simulink model "Opticflowtest"  (Simulink 7.6)
settings: Solver=ode45  StartTime=0.0  StopTime=inf  RelTol=1e-3
undefined symbols (not defined in the file or in its folder): Horn, none, Schunck, videoinput
libraries: imaqlib x1, dspstat3 x1, vipanalysis x1, simulink x1
settings Model: Creator=pacifist  LastModifiedBy=pacifist

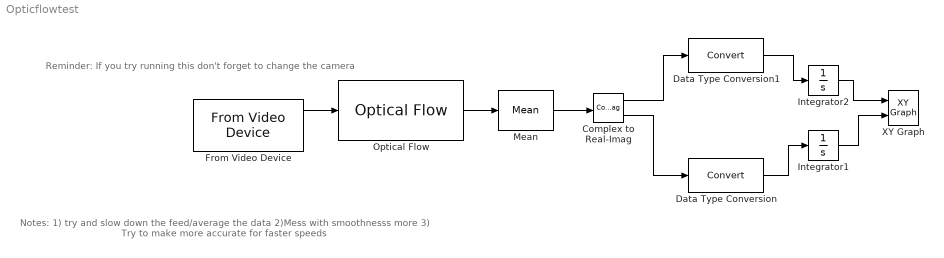
== system Opticflowtest ==
  note: Notes:
      | 1) try and slow down the feed/average the data
      | 2)Mess with smoothnesss more
      | 3) Try to make more accurate for faster speeds
  note: Reminder:
      | If you try running this don't forget to change the camera
  Complex to Real-Imag : ComplexToRealImag
  Data Type Conversion : DataTypeConversion
  Data Type Conversion1 : DataTypeConversion
  From Video Device : imaqlib/From Video Device  DialogController=imaqcreatedialog  DialogControllerArgs=DataTag1  DeviceMenu=linuxvideo 1 (UVC Camera (046d:0804))  Device=linuxvideo 1 (UVC Camera (046d:0804))  ObjConstructor=videoinput('linuxvideo', 1)  VideoFormatMenu=YUYV_160x120  VideoFormat=YUYV_160x120  VideoSource=Camera 1  ROIPosition=[0 0 120 160]  EnableHWTrigger=off  TriggerConfiguration=none/none  SampleTime=1/30  OutputPortsMode=Separate color signals  DataType=single  CanDoHWTrigger=no  ReturnedColorSpace=YCbCr  BlockHandle=2231.0004  ROIWidth=160  ROIHeight=120  ROIColumn=0  ROIRow=0  EngXMLPath=/usr/local/MATLAB/R2010b/toolbox/imaq/imaq/private  DevXMLPath=/usr/local/MATLAB/R2010b/toolbox/imaq/imaqadaptors/glnx86  EngLibPath=/usr/local/MATLAB/R2010b/toolbox/imaq/imaqblks/imaqmex/glnx86
  Integrator1 : Integrator  LimitOutput=on  UpperSaturationLimit=.01  LowerSaturationLimit=-.01
  Integrator2 : Integrator  LimitOutput=on  UpperSaturationLimit=.01  LowerSaturationLimit=-.01
  Mean : dspstat3/Mean  DialogController=dspDDGCreate  DialogControllerArgs=DataTag3  run=off  reset_popup=None  directionMode=Entire input  dimension=1  treatSBRowAsCol=on  roiEnable=off  roiType=Rectangles  roiPortion=Entire ROI  roiOutput=Individual statistics for each ROI  roiFlag=off  outputDataTypeStr=Inherit: Same as accumulator  outputLastDataTypeStr=Inherit: Same as accumulator  outputMin=[]  outputMax=[]  accumMode=Binary point scaling  accumWordLength=32  accumFracLength=0  accumDataTypeStr=fixdt([],32,0)  accumLastDataTypeStr=fixdt([],32,0)  roundingMode=Floor  overflowMode=off
  Optical Flow : vipanalysis/Optical Flow  DialogController=vipDDGCreate  DialogControllerArgs=DataTag4  SystemSampleTime=-1  method=Horn-Schunck  gradMethod=Difference filter [-1 1]  which2img=Current frame and N-th frame back  N=1  outVelForm=Horizontal and vertical components in complex form  lambda=5  stop_criteria=When maximum number of iterations is reached  maxAllowAbsDiff=eps  maxIter=10  numInports=3  sigmaS=1.5  sigmaW=1  eigTh=0.0039  discardNormalFlow=off  outputCurrentImage=off  prodOutputMode=Binary point scaling  prodOutputWordLength=32  prodOutputFracLength=20  outputMode=Binary point scaling  outputWordLength=32  outputFracLength=20  roundingMode=Nearest  overflowMode=on
      link override Optical Flow Estimation: which2img=Current frame and N-th frame back  outVelForm=Magnitude-squared
  XY Graph : simulink/Sinks/XY Graph  SystemSampleTime=-1  xmin=-.01  xmax=.01  ymin=-.01  ymax=.01  st=-1
  wires:
  Optical Flow/1 -> Mean/1
  From Video Device/1 -> Optical Flow/1
  Mean/1 -> Complex to Real-Imag/1
  Integrator2/1 -> XY Graph/1
  Integrator1/1 -> XY Graph/2
  Complex to Real-Imag/1 -> Data Type Conversion1/1
  Complex to Real-Imag/2 -> Data Type Conversion/1
  Data Type Conversion/1 -> Integrator1/1
  Data Type Conversion1/1 -> Integrator2/1
